simulink model "MPCNN"  (R2023a)
settings: Solver=ode1  StartTime=0.0  StopTime=inf  FixedStep=0.005  RelTol=1e-3  EnableMultiTasking=on
libraries: neural x20
(part 1 of 3)
settings Model: ExtModeTrigDuration=10000  Creator=XIJ62  LastModifiedBy=XIJ62
settings SolverCC: AlgebraicLoopSolver=TrustRegion  PositivePriorityOrder=on
settings DataIOCC: ReturnWorkspaceOutputs=off
settings DebuggingCC: UnconnectedInputMsg=warning  UnconnectedOutputMsg=warning  UnconnectedLineMsg=warning  ArithmeticOperatorsInVariantConditions=warning
settings ModelReferenceCC: EnableRefExpFcnMdlSchedulingChecks=on
settings SFSimCC: SimUseLocalCustomCode=off  CustomCodeUndefinedFunction=UseInterfaceOnly
settings RTWCC: Description=QUARC Win64 Target Using Toolchain  SystemTargetFile=quarc_win64.tlc  TemplateMakefile=quarc_default_tmf  RTWUseLocalCustomCode=off  Toolchain=QUARC win64 | nmake (64-bit Windows)  BuildConfiguration=Faster Runs  DLArmComputeVersion=19.05
settings CodeAppCC: StateflowObjectComments=on
settings STFCustomTargetCC: SystemTargetFile=quarc_win64.tlc
settings GRTTargetCC: ParMdlRefBuildCompliant=off  CompOptLevelCompliant=off  CombineOutputUpdateFcns=off  MatFileLogging=off  CPPClassGenCompliant=off  GRTInterface=on  ExtMode=on  ExtModeMexFile=quarc_comm
settings ConfigComp: CovMetricSettings=dswe

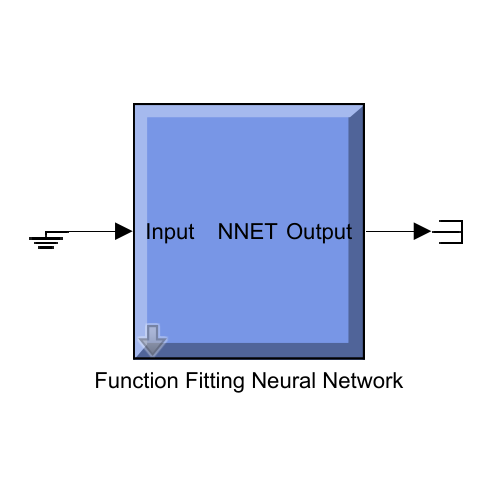
[thumbnail: Simulink's stored preview of the top-level diagram]
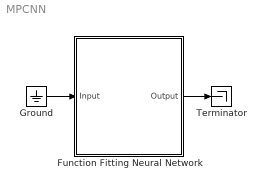
== system MPCNN ==
  Function Fitting Neural Network : Subsystem
      mask help: Function Fitting Neural Network
      mask Display: e = 0.06;c1 = [120 150 230]/255;c2 = ([120 150 230]+0)/383;c3 = ([120 150 230]+128)/383;patch([0 1 1 0],[0 0 1 1],c1);patch([0 1 1 1-e 1-e 0+e],[0 0 1 1-e 0+e 0+e],c2);patch([0 0 1 1-e 0+e 0+e],[0 1 1 1-e 1-e 0+e],c3);plot([0 1 1 0 0],[0 0 1 1 0]);fprintf('NNET');port_label('input',1,' Input');port_label('output',1,'Output ');
  Ground : Ground
  Terminator : Terminator
  wires:
  Function Fitting Neural Network/1(Output) -> Terminator/1
  Ground/1 -> Function Fitting Neural Network/1(Input)

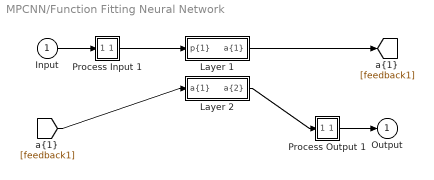
== system MPCNN/Function Fitting Neural Network ==
  Input : Inport  PortDimensions=124
      mask Display: e = 0.06;c1 = [120 230 180]/255;c2 = ([120 230 180]+0)/(256+128);c3 = ([120 230 180]+128)/(256+128);patch([0 1 1 0],[0 0 1 1],c1);patch([0 1 1 1-e 1-e 0+e],[0 0 1 1-e 0+e 0+e],c2);patch([0 0 1 1-e 0+e 0+e],[0 1 1 1-e 1-e 0+e],c3);plot([0 1 1 0 0],[0 0 1 1 0]);
  Layer 1 : Subsystem
      mask Display: e = 0.06;c1 = [120 150 230]/255;c2 = ([120 150 230]+0)/383;c3 = ([120 150 230]+128)/383;patch([0 1 1 0],[0 0 1 1],c1);patch([0 1 1 1-e 1-e 0+e],[0 0 1 1-e 0+e 0+e],c2);patch([0 0 1 1-e 0+e 0+e],[0 1 1 1-e 1-e 0+e],c3);plot([0 1 1 0 0],[0 0 1 1 0]);
  Layer 2 : Subsystem
      mask Display: e = 0.06;c1 = [120 150 230]/255;c2 = ([120 150 230]+0)/383;c3 = ([120 150 230]+128)/383;patch([0 1 1 0],[0 0 1 1],c1);patch([0 1 1 1-e 1-e 0+e],[0 0 1 1-e 0+e 0+e],c2);patch([0 0 1 1-e 0+e 0+e],[0 1 1 1-e 1-e 0+e],c3);plot([0 1 1 0 0],[0 0 1 1 0]);
  Process Input 1 : Subsystem
      mask Display: e = 0.06;c1 = [120 150 230]/255;c2 = ([120 150 230]+0)/383;c3 = ([120 150 230]+128)/383;patch([0 1 1 0],[0 0 1 1],c1);patch([0 1 1 1-e 1-e 0+e],[0 0 1 1-e 0+e 0+e],c2);patch([0 0 1 1-e 0+e 0+e],[0 1 1 1-e 1-e 0+e],c3);plot([0 1 1 0 0],[0 0 1 1 0]);
  Process Output 1 : Subsystem
      mask Display: e = 0.06;c1 = [120 150 230]/255;c2 = ([120 150 230]+0)/383;c3 = ([120 150 230]+128)/383;patch([0 1 1 0],[0 0 1 1],c1);patch([0 1 1 1-e 1-e 0+e],[0 0 1 1-e 0+e 0+e],c2);patch([0 0 1 1-e 0+e 0+e],[0 1 1 1-e 1-e 0+e],c3);plot([0 1 1 0 0],[0 0 1 1 0]);
  Output : Outport  InitialOutput=0
      mask Display: e = 0.06;c1 = [120 230 180]/255;c2 = ([120 230 180]+0)/(256+128);c3 = ([120 230 180]+128)/(256+128);patch([0 1 1 0],[0 0 1 1],c1);patch([0 1 1 1-e 1-e 0+e],[0 0 1 1-e 0+e 0+e],c2);patch([0 0 1 1-e 0+e 0+e],[0 1 1 1-e 1-e 0+e],c3);plot([0 1 1 0 0],[0 0 1 1 0]);
  wires:
  Input/1 -> Process Input 1/1(x)
  Process Output 1/1(y) -> Output/1
  Process Input 1/1(p) -> Layer 1/1("p{1}")
  Layer 1/1("a{1}") -> [feedback1]
  [feedback1] -> Layer 2/1("a{1} ")
  Layer 2/1("a{2}") -> Process Output 1/1(a)

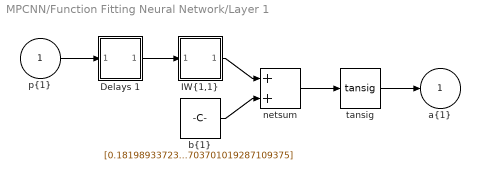
== system MPCNN/Function Fitting Neural Network/Layer 1 ==
  "p{1}" : Inport  PortDimensions=124
      mask Display: e = 0.06;c1 = [120 230 180]/255;c2 = ([120 230 180]+0)/(256+128);c3 = ([120 230 180]+128)/(256+128);patch([0 1 1 0],[0 0 1 1],c1);patch([0 1 1 1-e 1-e 0+e],[0 0 1 1-e 0+e 0+e],c2);patch([0 0 1 1-e 0+e 0+e],[0 1 1 1-e 1-e 0+e],c3);plot([0 1 1 0 0],[0 0 1 1 0]);
  Delays 1 : Subsystem
      mask Display: e = 0.06;c1 = [120 150 230]/255;c2 = ([120 150 230]+0)/383;c3 = ([120 150 230]+128)/383;patch([0 1 1 0],[0 0 1 1],c1);patch([0 1 1 1-e 1-e 0+e],[0 0 1 1-e 0+e 0+e],c2);patch([0 0 1 1-e 0+e 0+e],[0 1 1 1-e 1-e 0+e],c3);plot([0 1 1 0 0],[0 0 1 1 0]);disp('0');
  "IW{1,1}" : Subsystem
      mask Display: e = 0.06;c1 = [120 150 230]/255;c2 = ([120 150 230]+0)/383;c3 = ([120 150 230]+128)/383;patch([0 1 1 0],[0 0 1 1],c1);patch([0 1 1 1-e 1-e 0+e],[0 0 1 1-e 0+e 0+e],c2);patch([0 0 1 1-e 0+e 0+e],[0 1 1 1-e 1-e 0+e],c3);plot([0 1 1 0 0],[0 0 1 1 0]);disp('W');
  "b{1}" : Constant  Value=[0.181989337237214610087931987436604686081409454345703125;1.6578812832445108949031009615282528102397918701171875;-1.215359844012722678741056370199657976627349853515625;-0.0089788008202862333584359788574147387407720088958740234375;-0.00638555126426833437325303322040781495161354541778564453125;-1.01487854222639573009701052797026932239532470703125;0.324572918450551750613186641203355975449085235595703125;-0.7057379215684047579770776792429387569427490234375;-0.24488316305143043027925386923016048967838287353515625;0.0514385741610186852934560874928138218820095062255859375;2.168178946048700428406164064654149115085601806640625;-0.06099469593891877761127062740342807956039905548095703125;0.74420907551594350781698494756710715591907501220703125;0.6151289408296334304537822390557266771793365478515625;-1.88925559395558817499249926186166703701019287109375]
      mask Display: e = 0.06;c1 = [120 150 230]/255;c2 = ([120 150 230]+0)/383;c3 = ([120 150 230]+128)/383;patch([0 1 1 0],[0 0 1 1],c1);patch([0 1 1 1-e 1-e 0+e],[0 0 1 1-e 0+e 0+e],c2);patch([0 0 1 1-e 0+e 0+e],[0 1 1 1-e 1-e 0+e],c3);plot([0 1 1 0 0],[0 0 1 1 0]);disp('b');
  netsum : Sum  Inputs=2  InputSameDT=on  SaturateOnIntegerOverflow=on  OutDataTypeStr=Inherit: Same as first input
      mask Display: e = 0.06;c1 = [120 150 230]/255;c2 = ([120 150 230]+0)/383;c3 = ([120 150 230]+128)/383;patch([0 1 1 0],[0 0 1 1],c1);patch([0 1 1 1-e 1-e 0+e],[0 0 1 1-e 0+e 0+e],c2);patch([0 0 1 1-e 0+e 0+e],[0 1 1 1-e 1-e 0+e],c3);plot([0 1 1 0 0],[0 0 1 1 0]);disp('+');
  tansig : neural/Transfer Functions/tansig
  "a{1}" : Outport  InitialOutput=[0;0;0;0;0;0;0;0;0;0;0;0;0;0;0]
      mask Display: e = 0.06;c1 = [120 230 180]/255;c2 = ([120 230 180]+0)/(256+128);c3 = ([120 230 180]+128)/(256+128);patch([0 1 1 0],[0 0 1 1],c1);patch([0 1 1 1-e 1-e 0+e],[0 0 1 1-e 0+e 0+e],c2);patch([0 0 1 1-e 0+e 0+e],[0 1 1 1-e 1-e 0+e],c3);plot([0 1 1 0 0],[0 0 1 1 0]);
  wires:
  "p{1}"/1 -> Delays 1/1("p{1}")
  Delays 1/1("pd{1,1}") -> "IW{1,1}"/1("pd{1,1}")
  "IW{1,1}"/1("iz{1,1}") -> netsum/1
  "b{1}"/1 -> netsum/2
  netsum/1 -> tansig/1
  tansig/1 -> "a{1}"/1

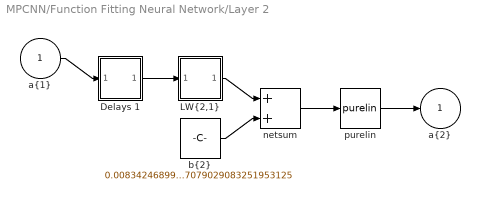
== system MPCNN/Function Fitting Neural Network/Layer 2 ==
  "a{1} " : Inport  PortDimensions=15
      mask Display: e = 0.06;c1 = [120 230 180]/255;c2 = ([120 230 180]+0)/(256+128);c3 = ([120 230 180]+128)/(256+128);patch([0 1 1 0],[0 0 1 1],c1);patch([0 1 1 1-e 1-e 0+e],[0 0 1 1-e 0+e 0+e],c2);patch([0 0 1 1-e 0+e 0+e],[0 1 1 1-e 1-e 0+e],c3);plot([0 1 1 0 0],[0 0 1 1 0]);
  Delays 1 : Subsystem
      mask Display: e = 0.06;c1 = [120 150 230]/255;c2 = ([120 150 230]+0)/383;c3 = ([120 150 230]+128)/383;patch([0 1 1 0],[0 0 1 1],c1);patch([0 1 1 1-e 1-e 0+e],[0 0 1 1-e 0+e 0+e],c2);patch([0 0 1 1-e 0+e 0+e],[0 1 1 1-e 1-e 0+e],c3);plot([0 1 1 0 0],[0 0 1 1 0]);disp('0');
  "LW{2,1}" : Subsystem
      mask Display: e = 0.06;c1 = [120 150 230]/255;c2 = ([120 150 230]+0)/383;c3 = ([120 150 230]+128)/383;patch([0 1 1 0],[0 0 1 1],c1);patch([0 1 1 1-e 1-e 0+e],[0 0 1 1-e 0+e 0+e],c2);patch([0 0 1 1-e 0+e 0+e],[0 1 1 1-e 1-e 0+e],c3);plot([0 1 1 0 0],[0 0 1 1 0]);disp('W');
  "b{2}" : Constant  Value=0.00834246899025244299796799651858236757107079029083251953125
      mask Display: e = 0.06;c1 = [120 150 230]/255;c2 = ([120 150 230]+0)/383;c3 = ([120 150 230]+128)/383;patch([0 1 1 0],[0 0 1 1],c1);patch([0 1 1 1-e 1-e 0+e],[0 0 1 1-e 0+e 0+e],c2);patch([0 0 1 1-e 0+e 0+e],[0 1 1 1-e 1-e 0+e],c3);plot([0 1 1 0 0],[0 0 1 1 0]);disp('b');
  netsum : Sum  Inputs=2  InputSameDT=on  SaturateOnIntegerOverflow=on  OutDataTypeStr=Inherit: Same as first input
      mask Display: e = 0.06;c1 = [120 150 230]/255;c2 = ([120 150 230]+0)/383;c3 = ([120 150 230]+128)/383;patch([0 1 1 0],[0 0 1 1],c1);patch([0 1 1 1-e 1-e 0+e],[0 0 1 1-e 0+e 0+e],c2);patch([0 0 1 1-e 0+e 0+e],[0 1 1 1-e 1-e 0+e],c3);plot([0 1 1 0 0],[0 0 1 1 0]);disp('+');
  purelin : neural/Transfer Functions/purelin
  "a{2}" : Outport  InitialOutput=0
      mask Display: e = 0.06;c1 = [120 230 180]/255;c2 = ([120 230 180]+0)/(256+128);c3 = ([120 230 180]+128)/(256+128);patch([0 1 1 0],[0 0 1 1],c1);patch([0 1 1 1-e 1-e 0+e],[0 0 1 1-e 0+e 0+e],c2);patch([0 0 1 1-e 0+e 0+e],[0 1 1 1-e 1-e 0+e],c3);plot([0 1 1 0 0],[0 0 1 1 0]);
  wires:
  "a{1} "/1 -> Delays 1/1("p{2}")
  Delays 1/1("pd{2,1}") -> "LW{2,1}"/1("ad{2,1}")
  "LW{2,1}"/1("lz{2,1}") -> netsum/1
  "b{2}"/1 -> netsum/2
  netsum/1 -> purelin/1
  purelin/1 -> "a{2}"/1

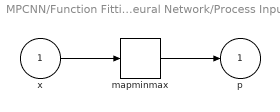
== system MPCNN/Function Fitting Neural Network/Process Input 1 ==
  x : Inport  PortDimensions=124
      mask Display: e = 0.06;c1 = [120 230 180]/255;c2 = ([120 230 180]+0)/(256+128);c3 = ([120 230 180]+128)/(256+128);patch([0 1 1 0],[0 0 1 1],c1);patch([0 1 1 1-e 1-e 0+e],[0 0 1 1-e 0+e 0+e],c2);patch([0 0 1 1-e 0+e 0+e],[0 1 1 1-e 1-e 0+e],c3);plot([0 1 1 0 0],[0 0 1 1 0]);
  mapminmax : neural/Processing Functions/mapminmax  xmin=[-1;-0.299999999999999988897769753748;-3;-3;-1.24990757156454845855364510498;-1.2498276166095072525763498561;-1.24984247004924498014588607475;-1.24946785011359029482491678209;-1.24972846531745029885485109844;-1.2499589844192109389098277461;-1.24999285595731923770301818877;-1.24998579918865582172315953358;-1.24996120406213639952852645365;-1.24992219265748705225860248902;-1.24996529150263158136624497274;-1.24982988052387367083895242104;-1.24991402347667790451168912114;-1.24985152022810774852246140654;-1.24988202967451345060112544161;-1.24982948670102422816796661209;-1.24948803538897745823987861513;-1.24974481749266819186061638902;-1.24992701939355965734534947842;-1.249657889622270756646571499;-1.24982303704838093594275960641;-1.24999520525608942556061720097;-1.24995479085048732947882399458;-1.24999458724969070289034789312;-1.24982509906070204941386236897;-1.24990350671498551271554333653;-1.24971951752336130070375475043;-1.24998950948509635061611788842;-1.24939591986022668912426070165;-1.24977163103468313920529908501;-1.24996205914323899044404697634;-1.249980991157562337789954654;-1.24987561175545880409742949269;-1.24989463284353674588089688768;-1.24990340220491091827170748729;-1.24996508826526464552841844124;-1.24989143304841765491630667384;-1.2494967764620423800181470142;-1.24971527115938219054669389152;-1.24946222592617184332652868761;-1.2499357188604918178498337511;-1.24995690126209901826825898752;-1.24979990591103096164715680061;-1.2494686345369696578444518309;-1.24950414920072527813488250104;-1.24989138140547195732210639108;-1.24981204265899670247108588228;-1.24990510867956738927375681669;-1.24999877730633168759766249423;-1.24992408393237042218970600516;-1.24989754594095003881193406414;-1.24992254913263334259454495623;-1.249857118823940460572430311;-1.24998864480785654151873131923;-1.24964674058967495362537647452;-1.24987347967563366957222115161;-1.24988676878550020177272017463;-1.24994670576710187326341383596;-1.24976063558361305538824126415;-1.2498120340489200508216072194;-1.24980617922834591482228461246;-1.2499507086046410808677364912;-1.24992397753888151434864539624;-1.24978489819746085842666616372;-1.2498570756762301670050874236;-1.24983296443682667664631935622;-1.24995457125754572125231334212;-1.24999424353456856096045157756;-1.24998071321759152141339654918;-1.24985523330533743191494977509;-1.24983049852676075808233235875;-1.24991264543752733651160724548;-1.24995404541268007037047027552;-1.24957790186414041677664954477;-1.24994429764166303797878754267;-1.24993925326003152420639707998;-1.24981847509914745231185406737;-1.24941104912168210461231865338;-1.24997748982900569458820427826;-1.24994927915737541468388371868;-1.24991793727101918598521024251;-1.249767535382716454606111256;-1.24980693398303221997025502787;-1.2496664851967731468818101348;-1.24928540168459623060925878235;-1.24961169209983258276963624667;-1.24980789242235545977166566445;-1.24997270178701347376204466855;-1.24992618869830263150788596249;-1.24936676121369316661002812907;-1.24995944119196678023797630885;-1.24966102464371076052884745877;-1.24981589056486463995554458961;-1.24999186050637978162569652341;-1.24989754109994199993138863647;-1.24972765599697077654184340645;-1.24989085443783864981526221527;-1.24984944029317346370078212203;-1.24999501253621936314175400184;-1.24993781965046824034004657733;-1.2499270538637379246438285918;-1.24986176699333007000802808761;-1.2498614430484324966386111555;-1.24999029879191181358066842222;-1.24985904929991376022258009471;-1.24946914735104974703006064374;-1.24960343441836574385206404258;-1.24991087926750710224155227479;-1.24985041975046762274814682314;-1.24996927203130692163313142373;-1.24989104639099157800785633299;-1.24975601797603097509181679925;-1.24982366654018228757649922045;-1.24994728484700057258294236817;-1.24993644872945641743910982768;-1.2499218979638790916197876868;-1.24991676629261894149180989189;-1.24987000557929439636950519343;-1.24978515504360609966738593357;-1.24990745183962781439390710148]  xmax=[1;0.299999999999999988897769753748;3;3;1.24993290011808877437715636916;1.24988774098404942236584247439;1.2498785514081247605133739853;1.24998104120053632470899174223;1.24993003693424498123931698501;1.24985000564343451401327911299;1.2499951269707305634426575125;1.24988593334113140542740438832;1.24985781393667982897000001685;1.24998629964217444765495201864;1.24949305409404676225904040621;1.24963074887824499015209767094;1.24999169820039446321402465401;1.24986918889539033727942296537;1.24996160358031405124279444863;1.24997747626961652755994691688;1.24997189642010519960990677646;1.24992816668042117100867471891;1.24994683203243539537652395666;1.24992417120550314280080783647;1.24999174515003419472236600996;1.2498906500268720520807619323;1.24997359414645581310310262779;1.24991125998736007929323932331;1.24971401445090535275994625408;1.24995964940233639239863805415;1.24996975151664901915182781522;1.24996106101056048132136311324;1.24995130084837224870852878666;1.24977702272797275284688112151;1.24998479129488426764282849035;1.24993862336965255721565881686;1.24981301198758298909297081991;1.24999870735858875647750210192;1.24999528020526540217360889073;1.24966084662959930895453908306;1.2499776059710159259452666447;1.24944375282499109403033799026;1.24988660546435514930863064365;1.24990610300701154855573804525;1.24985420341307174041389771446;1.24963956660906028162116854219;1.24956884456895034318790749239;1.24990103257889728638474480249;1.24997390433114841101769343368;1.24994008462113770363544063002;1.24995414670738735907207228593;1.24998048924572247031505867199;1.24974965468391063794229012274;1.24994259461455570203725073952;1.24983517090027884677283509518;1.24969264022565917926499423629;1.2499030974597538090620219009;1.24978816673849291163378438796;1.24974612630519299472098282422;1.24971814700864936042989938869;1.24970339418141929144212554093;1.2499838230084336920810983429;1.24976058197197881227680227312;1.24975041395571562219402039773;1.24993260757853974496356386226;1.24998004363441639341658628837;1.24993146661083365245303866686;1.24976532849516752676777286979;1.24999941875550701908537121199;1.24995830856610812276130673126;1.24992371061435658674554360914;1.24988993618517341133156151045;1.24985936666555597085448425787;1.24982200422980671561390408897;1.24984697284395007699231427978;1.24979337414610425227579071361;1.24999217793589956215782876825;1.2493446066460469623393692018;1.24973644329779887129916460253;1.24951162821853856144116434734;1.24976712766580577707031807222;1.24999672844367459845216217218;1.24983999687365265884864129475;1.24977037679454516805321873107;1.24997707928827272993999031314;1.24988388887457535503244798747;1.24996106994413835877821838949;1.24985624574675480147334383219;1.24999519234957201518909641891;1.24977714920688143251936708111;1.24964130429448339043574378593;1.2499379219180504207997728372;1.24996871753968941121115676651;1.24984252893770086956237719278;1.24985986477310095921211541281;1.24995627429188616019928304013;1.24991872401219339394629059825;1.24971624506533496301585728361;1.24999562704774502819304871082;1.24979129619207229850985640951;1.24997506406344349727532971883;1.24947433373726202177067534649;1.24982350894694294041187276889;1.24982522043818056189934395661;1.24986742332105738029213171103;1.24932453731611703418025172141;1.24952036296852320162997784792;1.24993394924269152213014422159;1.24971361381193402095846067823;1.24984919525934978778991535364;1.24977279038180233428079191071;1.2499508558159093674078121694;1.24993506349370386843133928778;1.24996836394404153836035220593;1.24984736740538426857938247849;1.24987540652380646477581649378;1.24989452507353027144176849106;1.24995939062978056455222031218;1.24991521344861844511342496844;1.24950303906439019741014817555;1.24999871424442288159184499818;1.2494230503150305366943939589;1.24991566390761210669779757154;1.24921542690342013415261135378]  ymin=-1  ymax=1
  p : Outport  PortDimensions=124
      mask Display: e = 0.06;c1 = [120 230 180]/255;c2 = ([120 230 180]+0)/(256+128);c3 = ([120 230 180]+128)/(256+128);patch([0 1 1 0],[0 0 1 1],c1);patch([0 1 1 1-e 1-e 0+e],[0 0 1 1-e 0+e 0+e],c2);patch([0 0 1 1-e 0+e 0+e],[0 1 1 1-e 1-e 0+e],c3);plot([0 1 1 0 0],[0 0 1 1 0]);
  wires:
  x/1 -> mapminmax/1
  mapminmax/1 -> p/1

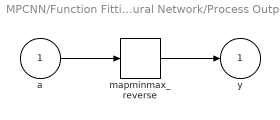
== system MPCNN/Function Fitting Neural Network/Process Output 1 ==
  a : Inport  PortDimensions=1
      mask Display: e = 0.06;c1 = [120 230 180]/255;c2 = ([120 230 180]+0)/(256+128);c3 = ([120 230 180]+128)/(256+128);patch([0 1 1 0],[0 0 1 1],c1);patch([0 1 1 1-e 1-e 0+e],[0 0 1 1-e 0+e 0+e],c2);patch([0 0 1 1-e 0+e 0+e],[0 1 1 1-e 1-e 0+e],c3);plot([0 1 1 0 0],[0 0 1 1 0]);
  mapminmax_reverse : neural/Processing Functions/mapminmax_reverse  xmin=-12.0000000000000248689957516035  xmax=12.0000000000000230926389122033  ymin=-1  ymax=1
  y : Outport  PortDimensions=1
      mask Display: e = 0.06;c1 = [120 230 180]/255;c2 = ([120 230 180]+0)/(256+128);c3 = ([120 230 180]+128)/(256+128);patch([0 1 1 0],[0 0 1 1],c1);patch([0 1 1 1-e 1-e 0+e],[0 0 1 1-e 0+e 0+e],c2);patch([0 0 1 1-e 0+e 0+e],[0 1 1 1-e 1-e 0+e],c3);plot([0 1 1 0 0],[0 0 1 1 0]);
  wires:
  a/1 -> mapminmax_reverse/1
  mapminmax_reverse/1 -> y/1

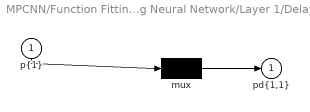
== system MPCNN/Function Fitting Neural Network/Layer 1/Delays 1 ==
  "p{1}" : Inport  PortDimensions=124
      mask Display: e = 0.06;c1 = [120 230 180]/255;c2 = ([120 230 180]+0)/(256+128);c3 = ([120 230 180]+128)/(256+128);patch([0 1 1 0],[0 0 1 1],c1);patch([0 1 1 1-e 1-e 0+e],[0 0 1 1-e 0+e 0+e],c2);patch([0 0 1 1-e 0+e 0+e],[0 1 1 1-e 1-e 0+e],c3);plot([0 1 1 0 0],[0 0 1 1 0]);
  mux : Mux  Inputs=1
      mask Display: e = 0.06;c1 = [120 150 230]/255;c2 = ([120 150 230]+0)/383;c3 = ([120 150 230]+128)/383;patch([0 1 1 0],[0 0 1 1],c1);patch([0 1 1 1-e 1-e 0+e],[0 0 1 1-e 0+e 0+e],c2);patch([0 0 1 1-e 0+e 0+e],[0 1 1 1-e 1-e 0+e],c3);plot([0 1 1 0 0],[0 0 1 1 0]);disp('Mux')
  "pd{1,1}" : Outport
      mask Display: e = 0.06;c1 = [120 230 180]/255;c2 = ([120 230 180]+0)/(256+128);c3 = ([120 230 180]+128)/(256+128);patch([0 1 1 0],[0 0 1 1],c1);patch([0 1 1 1-e 1-e 0+e],[0 0 1 1-e 0+e 0+e],c2);patch([0 0 1 1-e 0+e 0+e],[0 1 1 1-e 1-e 0+e],c3);plot([0 1 1 0 0],[0 0 1 1 0]);
  wires:
  "p{1}"/1 -> mux/1
  mux/1 -> "pd{1,1}"/1
